simulink model "ej4"  (R2023a)
settings: Solver=VariableStepAuto  StartTime=0.0  StopTime=10.0  RelTol=1e-3
model workspace (MAT data in the model file):
  a = 0.620196109442
  b = 0.468506025923
  c = 0.667399378458
  d = 0.443037974684
settings Model: Creator=santi  LastModifiedBy=santi

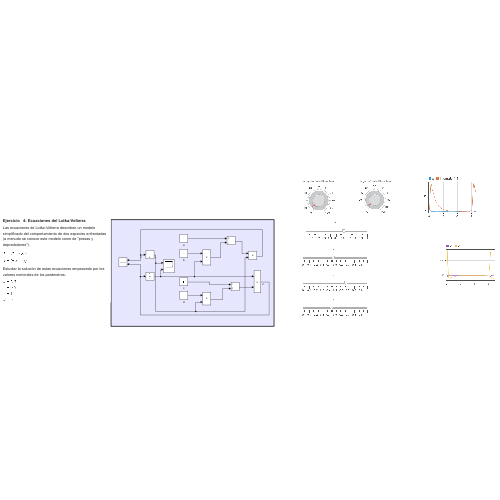
[thumbnail: Simulink's stored preview of the top-level diagram]
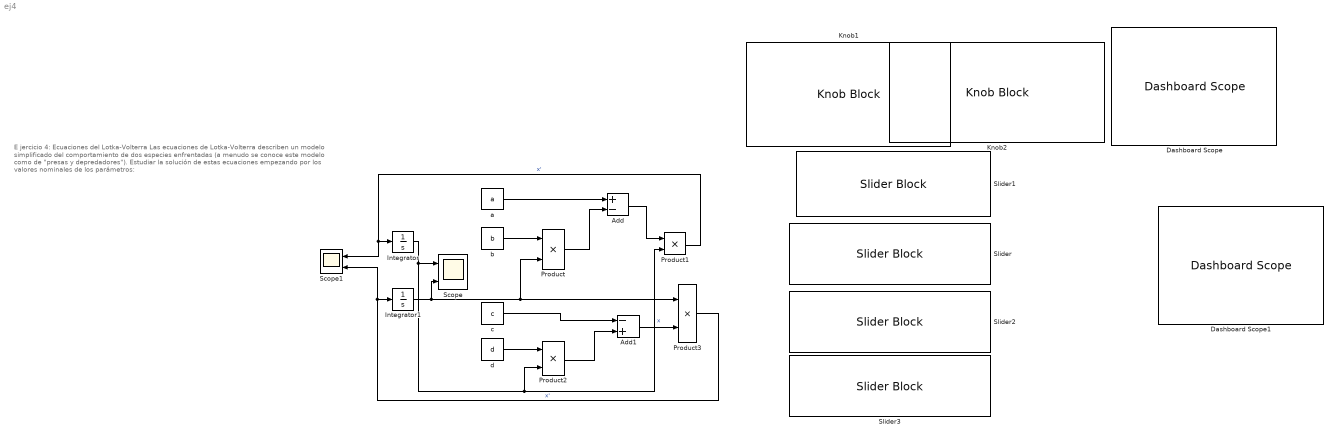
== system ej4 ==
  note: E jercicio 4: Ecuaciones del Lotka-Volterra
      | Las ecuaciones de Lotka-Volterra describen un modelo simplificado del comportamiento de dos especies enfrentadas (a menudo se conoce este modelo como de "presas y depredadores").
      |
      | Estudiar la solución de estas ecuaciones empezando por los valores nominales de los parámetros:
  Add : Sum  Inputs=+-
  Add1 : Sum  Inputs=-+
  Dashboard Scope : DashboardScope
  Dashboard Scope1 : DashboardScope
  Integrator : Integrator  InitialCondition=5
  Integrator1 : Integrator  InitialCondition=5
  Knob1 : KnobBlock
  Knob2 : KnobBlock
  Product{,1..3} (4 alike) : Product
  Scope : Scope  NumInputPorts=2
  Scope1 : Scope  NumInputPorts=2
  Slider{,1..3} (4 alike) : SliderBlock  ScaleMax=1
  a : Constant  Value=a
  b : Constant  Value=b
  c : Constant  Value=c
  d : Constant  Value=d
  wires:
  Integrator/1 -> Product1/2, Product2/2, Scope/1  "x"
  Integrator1/1 -> Scope/2, Product/2, Product3/1
  b/1 -> Product/1
  a/1 -> Add/1
  Product/1 -> Add/2
  Add/1 -> Product1/1
  Product1/1 -> Scope1/1, Integrator/1  "x'"
  d/1 -> Product2/1
  c/1 -> Add1/1
  Product2/1 -> Add1/2
  Add1/1 -> Product3/2
  Product3/1 -> Scope1/2, Integrator1/1  "x'"
